simulink model "DASD_B_Project_3"  (R2025b)
settings: Solver=FixedStepAuto  StartTime=0.0  StopTime=200  FixedStep=0.01  RelTol=1e-3
values from neighbouring files (symbols this model uses):
  a = 0.923    [VehicleParameters.m]
  a_max_acc = 2.0    (= 2)    [main.m]
  a_max_dec = -3.5    [main.m]
  ABS_parameters = [lower_acc; lower_slip; higher_acc; mean_acc; rise_rate; fall_rate]    [main.m]
  b = 1.376    [VehicleParameters.m]
  CMy = 0.1    [VehicleParameters.m]
  coeff = ones(1, fir_window) / fir_window    [main.m]
  Cx = 0.33    [VehicleParameters.m]
  Cz = 0.2    [VehicleParameters.m]
  dist0 = 100    [main.m]
  eta_t = 0.93    [VehicleParameters.m]
  f0 = 0.011    [VehicleParameters.m]
  g = 9.81    [VehicleParameters.m]
  gear_vec = i_g    [main.m]
  h = 2.7    [main.m]
  hG = 0.6    [VehicleParameters.m]
  I = kp / tau_virtual    (= 1.66666666667)    [main.m]
  i_f = 3.438    [VehicleParameters.m]
  i_g = [3.909 , 2.157 , 1.48 , 1.121 , 0.897]    [VehicleParameters.m]
  Je = 0.088    [VehicleParameters.m]
  Jt = 0.05    [VehicleParameters.m]
  Jw = 0.59    [VehicleParameters.m]
  K = 2.6e-8    (= 2.6e-08)    [VehicleParameters.m]
  l = a+b    (= 2.299)    [VehicleParameters.m]
  lambda = 0.8    [main.m]
  m = 1020    [VehicleParameters.m]
  mu_vec = road_cond{choice}    [main.m]
  n_shiftdown = 200    [main.m]
  n_shiftup = 500    [main.m]
  n_vec = n_vec_set{vec_choice}    [main.m]
  omega0 = v0/Re    [main.m]
  P = kp    (= 0.333333333333)    [main.m]
  Rc = Re    (= 0.279)    [VehicleParameters.m]
  ro = 1.2    [VehicleParameters.m]
  S = 2.04    [VehicleParameters.m]
  sigma_vec = sigma    [main.m]
  startingGear = 3    [main.m]
  t_pedalAct = 0.8    [VehicleParameters.m]
  t_shifting = 0.2    [VehicleParameters.m]
  T_vec = T_vec_set{vec_choice}    [main.m]
  tau_f = 1./i_f    (= 0.290866783013)    [VehicleParameters.m]
  Tc_max = 1.2*Te_max    (= 126)    [VehicleParameters.m]
  Traction = 1    [VehicleParameters.m]
  Ts = 0.01    [main.m]
  v0 = 30    [main.m]
  v_min_acc = 5.0    (= 5)    [main.m]
  v_set_min = 7.0    (= 7)    [main.m]
libraries: simulink x29, slpidlib x1
(part 1 of 2)
settings Model: Creator=Alberto  LastModifiedBy=denni
settings OptimizationCC: ReuseModelBlockBuffer=off
settings RTWCC: GPUComputeCapability=3.5

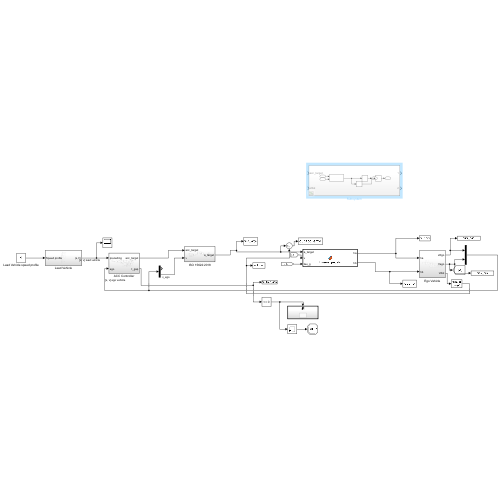
[thumbnail: Simulink's stored preview of the top-level diagram]
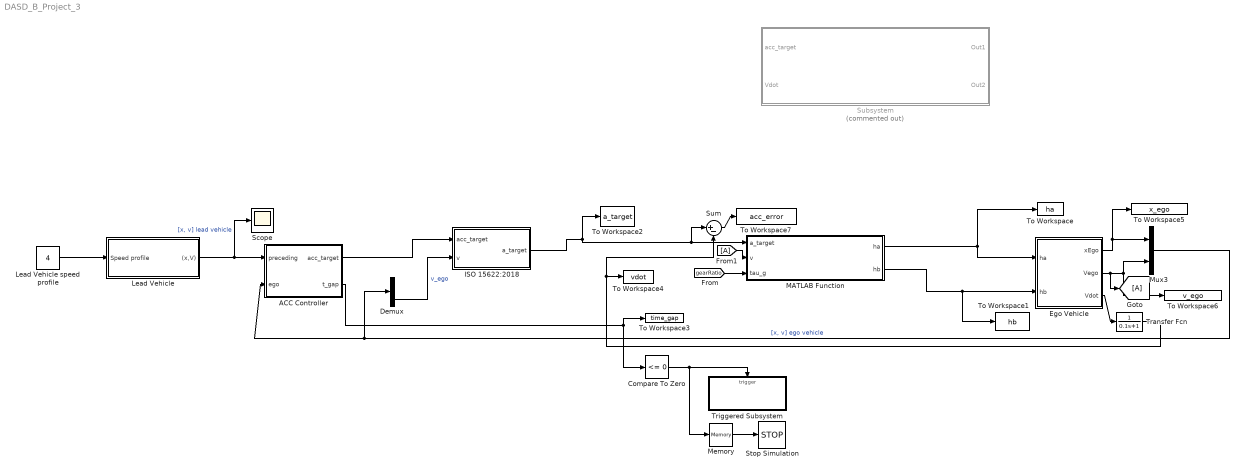
== system DASD_B_Project_3 ==
  ACC Controller : Subsystem
  Compare To Zero : simulink/Logic and Bit Operations/Compare To Zero  relop=<=  OutDataTypeStr=boolean
  Demux : Demux  Outputs=2
  Ego Vehicle : Subsystem
  From1 : From
  Goto : Goto
  ISO 15622:2018 : Subsystem
  Lead Vehicle : Subsystem
  Lead Vehicle speed profile : Constant  Value=4
  MATLAB Function : MATLAB Function  TreatAsAtomicUnit=on
  Memory : Memory
  Mux3 : Mux  Inputs=2
  Scope : Scope
      settings: ActiveDisplayYMinimum=0.0018281970394014024  ActiveDisplayYMaximum=37.912373720321341  DataLoggingVariableName=ScopeData13
  Stop Simulation : Stop
  Subsystem : Subsystem  Commented=on
  Sum : Sum  Inputs=|+-
  To Workspace : ToWorkspace  VariableName=ha  SaveFormat=Timeseries  SampleTime=-1
  To Workspace1 : ToWorkspace  VariableName=hb  SaveFormat=Timeseries  SampleTime=-1
  To Workspace2 : ToWorkspace  VariableName=a_target  SaveFormat=Timeseries  SampleTime=-1
  To Workspace3 : ToWorkspace  VariableName=time_gap  SaveFormat=Timeseries  SampleTime=-1
  To Workspace4 : ToWorkspace  VariableName=vdot  SaveFormat=Timeseries  SampleTime=-1
  To Workspace5 : ToWorkspace  VariableName=x_ego  SaveFormat=Timeseries  SampleTime=-1
  To Workspace6 : ToWorkspace  VariableName=v_ego  SaveFormat=Timeseries  SampleTime=-1
  To Workspace7 : ToWorkspace  VariableName=acc_error  SaveFormat=Timeseries  SampleTime=-1
  Transfer Fcn : TransferFcn  Denominator=[0.1 1]
  Triggered Subsystem : Subsystem  TreatAsAtomicUnit=on
  wires:
  Ego Vehicle/1(xEgo) -> To Workspace5/1, Mux3/1
  Ego Vehicle/2(Vego) -> Goto/1, To Workspace6/1, Mux3/2
  Mux3/1 -> Demux/1, ACC Controller/2(ego)  "[x, v] ego vehicle"
  Lead Vehicle/1((x,V)) -> Scope/1, ACC Controller/1(preceding)  "[x, v] lead vehicle"
  Lead Vehicle speed profile/1 -> Lead Vehicle/1(Speed profile)
  Memory/1 -> Stop Simulation/1
  Compare To Zero/1 -> Triggered Subsystem/Trigger, Memory/1
  ACC Controller/2(t_gap) -> To Workspace3/1, Compare To Zero/1
  Demux/2 -> ISO 15622:2018/2(v)  "v_ego"
  ACC Controller/1(acc_target) -> ISO 15622:2018/1(acc_target)
  ISO 15622:2018/1(a_target) -> To Workspace2/1, Sum/1, MATLAB Function/1(a_target)
  Ego Vehicle/3(Vdot) -> Transfer Fcn/1
  Transfer Fcn/1 -> To Workspace4/1, Sum/2
  [gearRatio] -> MATLAB Function/3(tau_g)
  MATLAB Function/1(ha) -> Ego Vehicle/1(ha), To Workspace/1
  MATLAB Function/2(hb) -> To Workspace1/1, Ego Vehicle/2(hb)
  Sum/1 -> To Workspace7/1
  From1/1 -> MATLAB Function/2(v)

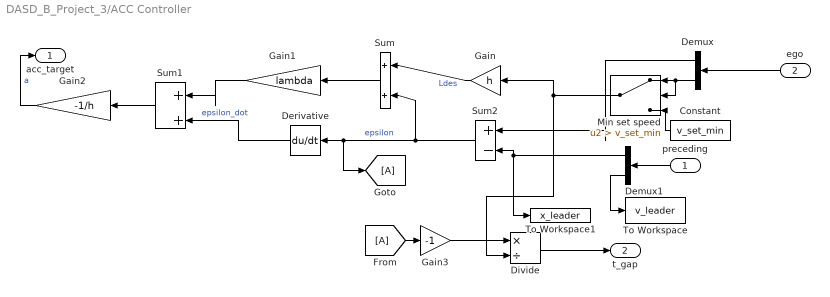
== system DASD_B_Project_3/ACC Controller ==
  preceding : Inport
  ego : Inport  Port=2
  Constant : Constant  Value=v_set_min
  Demux : Demux  Outputs=2
  Demux1 : Demux  Outputs=2
  Derivative : Derivative  CoefficientInTFapproximation=0.05
  Divide : Product  Inputs=*/
  From : From
  Gain : Gain  Gain=h
  Gain1 : Gain  Gain=lambda
  Gain2 : Gain  Gain=-1/h
  Gain3 : Gain  Gain=-1
  Goto : Goto
  Min set speed : Switch  Criteria=u2 > Threshold  Threshold=v_set_min  SaturateOnIntegerOverflow=off  InputSameDT=off
  Sum : Sum  Inputs=|++
  Sum1 : Sum  Inputs=|++
  Sum2 : Sum  Inputs=|+-
  To Workspace : ToWorkspace  VariableName=v_leader  SaveFormat=Timeseries  SampleTime=-1
  To Workspace1 : ToWorkspace  VariableName=x_leader  SaveFormat=Timeseries  SampleTime=-1
  acc_target : Outport
  t_gap : Outport  Port=2
  wires:
  Sum1/1 -> Gain2/1
  Sum/1 -> Gain1/1
  Gain2/1 -> acc_target/1  "a"
  Sum2/1 -> Sum/2, Goto/1, Derivative/1  "epsilon"
  Gain1/1 -> Sum1/1
  Gain/1 -> Sum/1  "Ldes"
  Derivative/1 -> Sum1/2  "epsilon_dot"
  ego/1 -> Demux/1
  preceding/1 -> Demux1/1
  Demux1/1 -> To Workspace1/1, Sum2/2
  Demux/1 -> Sum2/1
  Divide/1 -> t_gap/1
  From/1 -> Gain3/1
  Gain3/1 -> Divide/1
  Demux/2 -> Min set speed/2, Min set speed/1
  Min set speed/1 -> Divide/2, Gain/1
  Constant/1 -> Min set speed/3
  Demux1/2 -> To Workspace/1

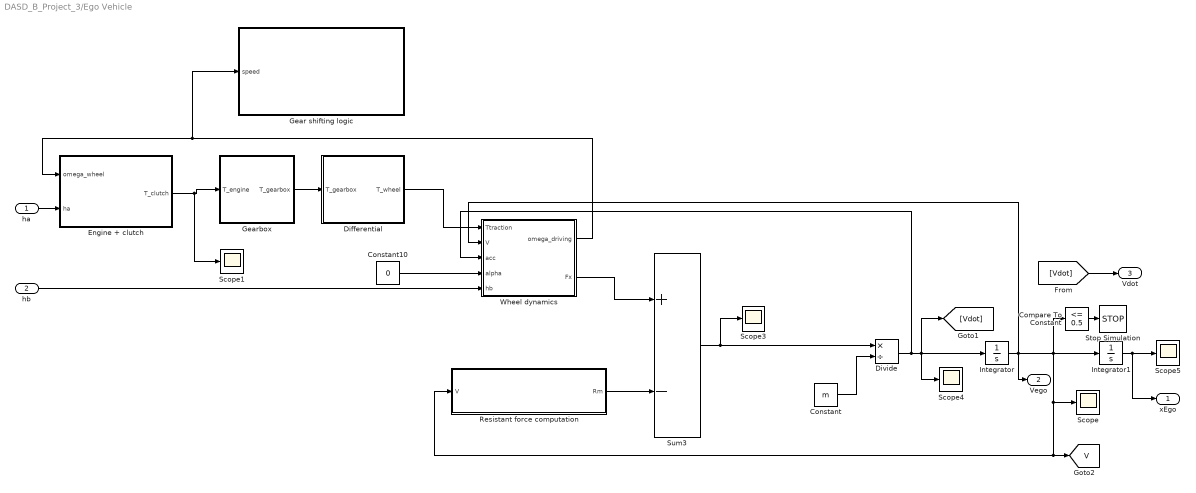
== system DASD_B_Project_3/Ego Vehicle ==
  ha : Inport
  hb : Inport  Port=2
  Compare To Constant : simulink/Logic and Bit Operations/Compare To Constant  relop=<=  const=0.5  OutDataTypeStr=boolean
  Constant : Constant  Value=m
  Constant10 : Constant  Value=0
  Differential : Subsystem
  Divide : Product  Inputs=*/
  Engine + clutch : Subsystem
  Gear shifting logic : Subsystem
  Gearbox : Subsystem
  Integrator : Integrator  InitialCondition=v0  UpperSaturationLimit=25  LowerSaturationLimit=5
  Integrator1 : Integrator
  Resistant force computation : Subsystem
  Scope{,1,3..5} (5 alike) : Scope
      Scope settings: ActiveDisplayYMinimum=2.5  ActiveDisplayYMaximum=26.27451
      Scope1 settings: ActiveDisplayYMinimum=-25.26926  ActiveDisplayYMaximum=122.58929  DataLoggingVariableName=ScopeData3
      Scope3 settings: ActiveDisplayYMinimum=-5116.83669  ActiveDisplayYMaximum=1269.91233  DataLoggingVariableName=ScopeData3
      Scope4 settings: ActiveDisplayYMinimum=-12.28873  ActiveDisplayYMaximum=11.6121  DataLoggingVariableName=ScopeData4
      Scope5 settings: ActiveDisplayYMinimum=969.20791  ActiveDisplayYMaximum=3277.1288
  Stop Simulation : Stop
  Sum3 : Sum  Inputs=+-
  Wheel dynamics : Subsystem
  xEgo : Outport
  Vego : Outport  Port=2
  Vdot : Outport  Port=3
  tag scope: V=global
  wires:
  Integrator/1 -> Wheel dynamics/2(V), Vego/1, Compare To Constant/1, [V], Resistant force computation/1(V), Scope/1, Integrator1/1
  Sum3/1 -> Scope3/1, Divide/1
  Compare To Constant/1 -> Stop Simulation/1
  Integrator1/1 -> xEgo/1, Scope5/1
  Divide/1 -> Wheel dynamics/3(acc), [Vdot], Scope4/1, Integrator/1
  Constant/1 -> Divide/2
  Resistant force computation/1(Rm) -> Sum3/2
  ha/1 -> Engine + clutch/2(ha)
  hb/1 -> Wheel dynamics/5(hb)
  Engine + clutch/1(T_clutch) -> Scope1/1, Gearbox/1(T_engine)
  Gearbox/1(T_gearbox) -> Differential/1(T_gearbox)
  Wheel dynamics/2(Fx) -> Sum3/1
  Differential/1(T_wheel) -> Wheel dynamics/1(Ttraction)
  Constant10/1 -> Wheel dynamics/4(alpha)
  Wheel dynamics/1(omega_driving) -> Gear shifting logic/1(speed), Engine + clutch/1(omega_wheel)
  [Vdot] -> Vdot/1

== system DASD_B_Project_3/ISO 15622:2018 ==
  acc_target : Inport
  v : Inport  Port=2
  Constant : Constant  Value=-3.5
  Constant1 : Constant  Value=0
  FIR filter for average acc evaluation : DiscreteFir  Coefficients=coeff
  Jerk Rate Limiter : RateLimiter  RisingSlewLimit=Inf  FallingSlewLimit=-2.5  SampleTimeMode=inherited
  Min : MinMax  Inputs=2
  Saturation : Saturate  UpperLimit=a_max_acc  LowerLimit=a_max_dec
  Scope : Scope
      settings: ActiveDisplayYMinimum=-37.751997370602687  ActiveDisplayYMaximum=46.44974892272235  DataLoggingVariableName=ScopeData12
  Switch : Switch  Criteria=u2 > Threshold  Threshold=a_max_dec  SaturateOnIntegerOverflow=off  InputSameDT=off
  Switch1 : Switch  Criteria=u2 > Threshold  Threshold=v_min_acc  SaturateOnIntegerOverflow=off  InputSameDT=off
  a_target : Outport
  wires:
  FIR filter for average acc evaluation/1 -> Switch/2
  Switch/1 -> Jerk Rate Limiter/1
  Switch1/1 -> Switch/1, FIR filter for average acc evaluation/1
  Jerk Rate Limiter/1 -> Scope/1, Saturation/1
  v/1 -> Switch1/2
  acc_target/1 -> Min/2, Switch1/1
  Min/1 -> Switch1/3
  Constant1/1 -> Min/1
  Constant/1 -> Switch/3
  Saturation/1 -> a_target/1

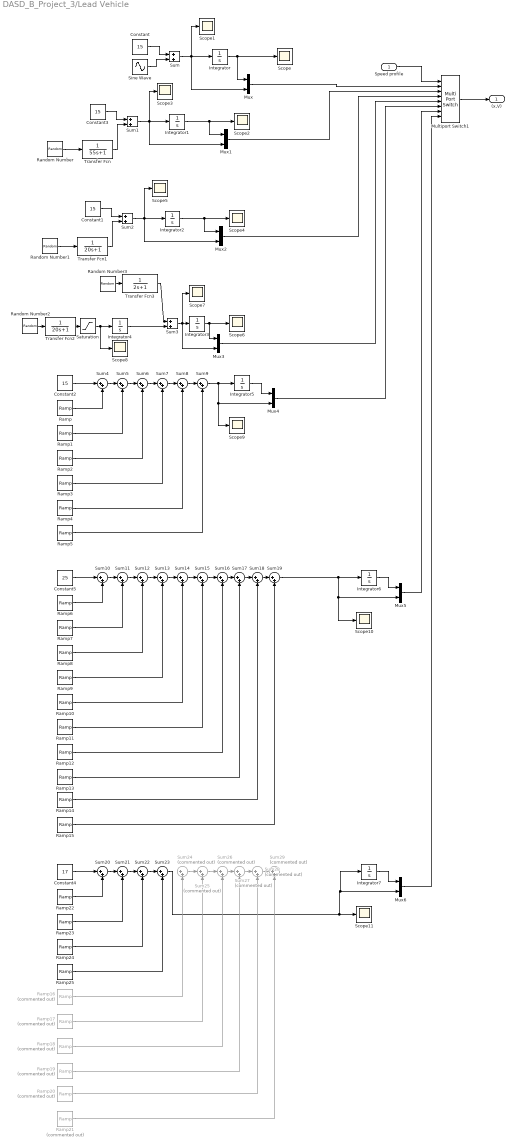
== system DASD_B_Project_3/Lead Vehicle ==
  Speed profile : Inport
  Constant{,1..3} (4 alike) : Constant  Value=15
  Constant4 : Constant  Value=17
  Constant5 : Constant  Value=25
  Integrator{,1..3,5..7} (7 alike) : Integrator  InitialCondition=dist0
  Integrator4 : Integrator  InitialCondition=15  LimitOutput=on  UpperSaturationLimit=27  LowerSaturationLimit=5
  Multiport Switch1 : MultiPortSwitch  Inputs=7  SaturateOnIntegerOverflow=off  InputSameDT=off
  Mux{,1..6} (7 alike) : Mux  Inputs=2
  Ramp : simulink/Sources/Ramp  slope=4  start=85  InitialOutput=0
  Ramp1 : simulink/Sources/Ramp  slope=-4  start=86.5  InitialOutput=0
  Ramp10 : simulink/Sources/Ramp  slope=1  start=105  InitialOutput=0
  Ramp11 : simulink/Sources/Ramp  slope=-1  start=120.3  InitialOutput=0
  Ramp12 : simulink/Sources/Ramp  slope=-15  start=150  InitialOutput=0
  Ramp13 : simulink/Sources/Ramp  slope=15  start=151.5  InitialOutput=0
  Ramp14 : simulink/Sources/Ramp  slope=8  start=165  InitialOutput=0
  Ramp15 : simulink/Sources/Ramp  slope=-8  start=167.8  InitialOutput=0
  Ramp16 : simulink/Sources/Ramp  Commented=on  slope=1  start=105  InitialOutput=0
  Ramp17 : simulink/Sources/Ramp  Commented=on  slope=-1  start=120.3  InitialOutput=0
  Ramp18 : simulink/Sources/Ramp  Commented=on  slope=-15  start=150  InitialOutput=0
  Ramp19 : simulink/Sources/Ramp  Commented=on  slope=15  start=151.5  InitialOutput=0
  Ramp2 : simulink/Sources/Ramp  slope=-12  start=150  InitialOutput=0
  Ramp20 : simulink/Sources/Ramp  Commented=on  slope=8  start=165  InitialOutput=0
  Ramp21 : simulink/Sources/Ramp  Commented=on  slope=-8  start=167.8  InitialOutput=0
  Ramp22 : simulink/Sources/Ramp  slope=-1  start=20  InitialOutput=0
  Ramp23 : simulink/Sources/Ramp  slope=1  start=30  InitialOutput=0
  Ramp24 : simulink/Sources/Ramp  slope=5  start=230  InitialOutput=0
  Ramp25 : simulink/Sources/Ramp  slope=-5  start=233  InitialOutput=0
  Ramp3 : simulink/Sources/Ramp  slope=12  start=151  InitialOutput=0
  Ramp4 : simulink/Sources/Ramp  slope=3  start=250  InitialOutput=0
  Ramp5 : simulink/Sources/Ramp  slope=-3  start=255  InitialOutput=0
  Ramp6 : simulink/Sources/Ramp  slope=-13  start=85  InitialOutput=0
  Ramp7 : simulink/Sources/Ramp  slope=13  start=86.6  InitialOutput=0
  Ramp8 : simulink/Sources/Ramp  slope=5  start=92  InitialOutput=0
  Ramp9 : simulink/Sources/Ramp  slope=-5  start=93.1  InitialOutput=0
  Random Number : RandomNumber  Variance=20  Seed=23564  SampleTime=5
  Random Number1 : RandomNumber  Variance=35  Seed=23564  SampleTime=1
  Random Number2 : RandomNumber  Variance=3  Seed=23564  SampleTime=2
  Random Number3 : RandomNumber  Variance=3  Seed=23564  SampleTime=2
  Saturation : Saturate  UpperLimit=5  LowerLimit=-5
  Scope{,1..11} (12 alike) : Scope
      Scope settings: ActiveDisplayYMinimum=62.13005  ActiveDisplayYMaximum=440.82954
      Scope1 settings: ActiveDisplayYMinimum=9.90107  ActiveDisplayYMaximum=19.94712  DataLoggingVariableName=ScopeData2
      Scope10 settings: ActiveDisplayYMinimum=-0.3125  ActiveDisplayYMaximum=27.8125  DataLoggingVariableName=ScopeData20
      Scope11 settings: ActiveDisplayYMinimum=5.125  ActiveDisplayYMaximum=23.875
      Scope2 settings: ActiveDisplayYMinimum=128.26697  ActiveDisplayYMaximum=160.50679  DataLoggingVariableName=ScopeData3
      Scope3 settings: ActiveDisplayYMinimum=13.6719  ActiveDisplayYMaximum=16.88686  DataLoggingVariableName=ScopeData4
      Scope4 settings: ActiveDisplayYMinimum=128.26697  ActiveDisplayYMaximum=160.50679  DataLoggingVariableName=ScopeData14
      Scope5 settings: ActiveDisplayYMinimum=12.15734  ActiveDisplayYMaximum=17.04494  DataLoggingVariableName=ScopeData15
      Scope6 settings: ActiveDisplayYMinimum=128.26697  ActiveDisplayYMaximum=160.50679  DataLoggingVariableName=ScopeData16
      Scope7 settings: ActiveDisplayYMinimum=-2.38071  ActiveDisplayYMaximum=32.83051  DataLoggingVariableName=ScopeData17
      Scope8 settings: ActiveDisplayYMinimum=-0.8596  ActiveDisplayYMaximum=0.81866  DataLoggingVariableName=ScopeData18
      Scope9 settings: ActiveDisplayYMinimum=7.125  ActiveDisplayYMaximum=25.875  DataLoggingVariableName=ScopeData19
  Sine Wave : Sin  Amplitude=5  SampleTime=0
  Sum{,1..3} (4 alike) : Sum
  Sum{4..23} (20 alike) : Sum  Inputs=|++
  Sum{24..29} (6 alike) : Sum  Commented=on  Inputs=|++
  Transfer Fcn : TransferFcn  Denominator=[55 1]
  Transfer Fcn1 : TransferFcn  Denominator=[20 1]
  Transfer Fcn2 : TransferFcn  Denominator=[20 1]
  Transfer Fcn3 : TransferFcn  Denominator=[2 1]
  (x,V) : Outport
  wires:
  Mux/1 -> Multiport Switch1/2
  Integrator/1 -> Scope/1, Mux/1
  Speed profile/1 -> Multiport Switch1/1
  Sum1/1 -> Integrator1/1, Mux1/2, Scope3/1
  Mux1/1 -> Multiport Switch1/3
  Transfer Fcn/1 -> Sum1/2
  Random Number/1 -> Transfer Fcn/1
  Constant/1 -> Sum/1
  Sine Wave/1 -> Sum/2
  Sum/1 -> Mux/2, Scope1/1, Integrator/1
  Integrator1/1 -> Mux1/1, Scope2/1
  Constant3/1 -> Sum1/1
  Multiport Switch1/1 -> (x,V)/1
  Constant1/1 -> Sum2/1
  Integrator2/1 -> Scope4/1, Mux2/1
  Random Number1/1 -> Transfer Fcn1/1
  Transfer Fcn1/1 -> Sum2/2
  Sum2/1 -> Integrator2/1, Scope5/1, Mux2/2
  Mux2/1 -> Multiport Switch1/4
  Mux3/1 -> Multiport Switch1/5
  Integrator4/1 -> Sum3/2
  Integrator3/1 -> Mux3/1, Scope6/1
  Saturation/1 -> Scope8/1, Integrator4/1
  Random Number2/1 -> Transfer Fcn2/1
  Transfer Fcn2/1 -> Saturation/1
  Sum3/1 -> Integrator3/1, Mux3/2, Scope7/1
  Random Number3/1 -> Transfer Fcn3/1
  Transfer Fcn3/1 -> Sum3/1
  Constant2/1 -> Sum4/1
  Ramp/1 -> Sum4/2
  Sum4/1 -> Sum5/1
  Ramp1/1 -> Sum5/2
  Sum5/1 -> Sum6/1
  Sum6/1 -> Sum7/1
  Ramp2/1 -> Sum6/2
  Ramp3/1 -> Sum7/2
  Sum7/1 -> Sum8/1
  Sum8/1 -> Sum9/1
  Ramp4/1 -> Sum8/2
  Ramp5/1 -> Sum9/2
  Sum9/1 -> Integrator5/1, Scope9/1, Mux4/2
  Integrator5/1 -> Mux4/1
  Mux4/1 -> Multiport Switch1/6
  Ramp6/1 -> Sum10/2
  Sum14/1 -> Sum15/1
  Ramp10/1 -> Sum14/2
  Sum10/1 -> Sum11/1
  Ramp9/1 -> Sum13/2
  Ramp8/1 -> Sum12/2
  Constant5/1 -> Sum10/1
  Ramp7/1 -> Sum11/2
  Sum12/1 -> Sum13/1
  Ramp11/1 -> Sum15/2
  Sum11/1 -> Sum12/1
  Sum13/1 -> Sum14/1
  Ramp13/1 -> Sum17/2
  Ramp12/1 -> Sum16/2
  Sum15/1 -> Sum16/1
  Sum16/1 -> Sum17/1
  Integrator6/1 -> Mux5/1
  Mux5/1 -> Multiport Switch1/7
  Sum17/1 -> Sum18/1
  Sum18/1 -> Sum19/1
  Ramp14/1 -> Sum18/2
  Ramp15/1 -> Sum19/2
  Sum19/1 -> Integrator6/1, Mux5/2, Scope10/1
  Sum23/1 -> Integrator7/1, Mux6/2, Scope11/1
  Sum25/1 -> Sum26/1
  Sum24/1 -> Sum25/1
  Sum28/1 -> Sum29/1
  Mux6/1 -> Multiport Switch1/8
  Ramp21/1 -> Sum29/2
  Ramp23/1 -> Sum21/2
  Ramp20/1 -> Sum28/2
  Ramp17/1 -> Sum25/2
  Ramp19/1 -> Sum27/2
  Sum20/1 -> Sum21/1
  Sum22/1 -> Sum23/1
  Constant4/1 -> Sum20/1
  Sum27/1 -> Sum28/1
  Ramp16/1 -> Sum24/2
  Integrator7/1 -> Mux6/1
  Ramp22/1 -> Sum20/2
  Ramp24/1 -> Sum22/2
  Ramp25/1 -> Sum23/2
  Ramp18/1 -> Sum26/2
  Sum26/1 -> Sum27/1
  Sum21/1 -> Sum22/1

== system DASD_B_Project_3/Subsystem ==
  acc_target : Inport
  Vdot : Inport  Port=2
  Abs : Abs  SaturateOnIntegerOverflow=off
  PI controller : Subsystem
  Saturation1 : Saturate  UpperLimit=1  LowerLimit=0
  Saturation2 : Saturate  UpperLimit=0  LowerLimit=-1
  Out1 : Outport
  Out2 : Outport  Port=2
  wires:
  Saturation1/1 -> Out1/1
  PI controller/1(a_target) -> Saturation2/1, Saturation1/1
  Saturation2/1 -> Abs/1
  Abs/1 -> Out2/1
  acc_target/1 -> PI controller/1(acc_target)
  Vdot/1 -> PI controller/2(Vdot)

== system DASD_B_Project_3/Triggered Subsystem ==
  Trigger : TriggerPort  VariantControl=(inherit)
  MATLAB Function : MATLAB Function  TreatAsAtomicUnit=on

== system DASD_B_Project_3/Ego Vehicle/Differential ==
  T_gearbox : Inport
  Gain3 : Gain  Gain=0.5*i_f
  T_wheel : Outport
  wires:
  T_gearbox/1 -> Gain3/1
  Gain3/1 -> T_wheel/1

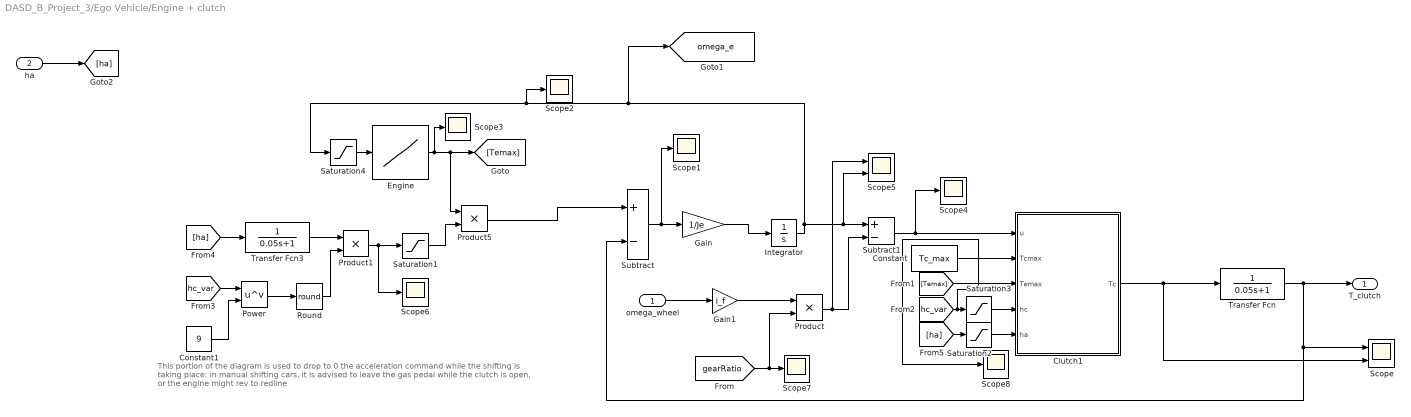
== system DASD_B_Project_3/Ego Vehicle/Engine + clutch ==
  note: This portion of the diagram is used to drop to 0 the acceleration command while the shifting is taking place: in manual shifting cars, it is advised to leave the gas pedal while the clutch is open, or the engine might rev to redline
  omega_wheel : Inport
  ha : Inport  Port=2
  Clutch1 : MATLAB Function  TreatAsAtomicUnit=on
  Constant : Constant  Value=Tc_max
  Constant1 : Constant  Value=9
  Engine : Lookup_n-D  NumberOfTableDimensions=1  BreakpointsForDimension1=n_vec  Table=T_vec  InternalRulePriority=Speed  RndMeth=Simplest
  Gain : Gain  Gain=1/Je
  Gain1 : Gain  Gain=i_f
  Integrator : Integrator  InitialCondition=omega0*i_g(5)*i_f
  Power : Math  Operator=pow
  Product : Product
  Product1 : Product
  Product5 : Product
  Round : Rounding  Operator=round
  Saturation1 : Saturate  UpperLimit=1  LowerLimit=0
  Saturation2 : Saturate  UpperLimit=1  LowerLimit=0
  Saturation3 : Saturate  UpperLimit=1  LowerLimit=0
  Saturation4 : Saturate  UpperLimit=600  LowerLimit=0
  Scope : Scope  NumInputPorts=2
      settings: ActiveDisplayYMinimum=-375  ActiveDisplayYMaximum=375  DataLoggingVariableName=ScopeData11
  Scope{1..4,6..8} (7 alike) : Scope
      Scope1 settings: ActiveDisplayYMinimum=-1.4800422611786087E+307  ActiveDisplayYMaximum=1.6444914013095649E+306  DataLoggingVariableName=ScopeData5
      Scope2 settings: ActiveDisplayYMinimum=-234.98976  ActiveDisplayYMaximum=2163.66995  DataLoggingVariableName=ScopeData6
      Scope3 settings: ActiveDisplayYMinimum=48.8411  ActiveDisplayYMaximum=110.12711  DataLoggingVariableName=ScopeData7
      Scope4 settings: ActiveDisplayYMinimum=-233.77506  ActiveDisplayYMaximum=296.88623  DataLoggingVariableName=ScopeData9
      Scope6 settings: ActiveDisplayYMinimum=-1  ActiveDisplayYMaximum=1
      Scope7 settings: ActiveDisplayYMinimum=3.85912  ActiveDisplayYMaximum=3.95022  DataLoggingVariableName=ScopeData2
      Scope8 settings: ActiveDisplayYMinimum=-0.11944  ActiveDisplayYMaximum=1.12438  DataLoggingVariableName=ScopeData2
  Scope5 : Scope  NumInputPorts=2
      settings: ActiveDisplayYMinimum=-194.18031  ActiveDisplayYMaximum=721.01575  DataLoggingVariableName=ScopeData10
  Subtract : Sum  Inputs=+-
  Subtract1 : Sum  Inputs=+-
  Transfer Fcn : TransferFcn  Denominator=[0.05 1]
  Transfer Fcn3 : TransferFcn  Denominator=[0.05 1]
  T_clutch : Outport
  tag scope: omega_e=global
  wires:
  Engine/1 -> Scope3/1, [Temax], Product5/1
  Product5/1 -> Subtract/1
  Saturation1/1 -> Product5/2
  Subtract/1 -> Scope1/1, Gain/1
  Gain/1 -> Integrator/1
  omega_wheel/1 -> Gain1/1
  Gain1/1 -> Product/1
  [gearRatio] -> Product/2, Scope7/1
  Product/1 -> Scope5/1, Subtract1/2
  Subtract1/1 -> Clutch1/1(u), Scope4/1
  Constant/1 -> Clutch1/2(Tcmax)
  [Temax] -> Clutch1/3(Temax)
  Transfer Fcn/1 -> Subtract/2, Scope/1, T_clutch/1
  Saturation3/1 -> Clutch1/4(hc)
  [hc_var] -> Scope8/1, Saturation3/1
  [ha] -> Saturation2/1
  Saturation2/1 -> Clutch1/5(ha)
  Integrator/1 -> [omega_e], Saturation4/1, Scope2/1, Scope5/2, Subtract1/1
  Transfer Fcn3/1 -> Product1/1
  Product1/1 -> Scope6/1, Saturation1/1
  Round/1 -> Product1/2
  [hc_var] -> Power/1
  Power/1 -> Round/1
  Constant1/1 -> Power/2
  Clutch1/1(Tc) -> Scope/2, Transfer Fcn/1
  Saturation4/1 -> Engine/1
  ha/1 -> [ha]
  [ha] -> Transfer Fcn3/1

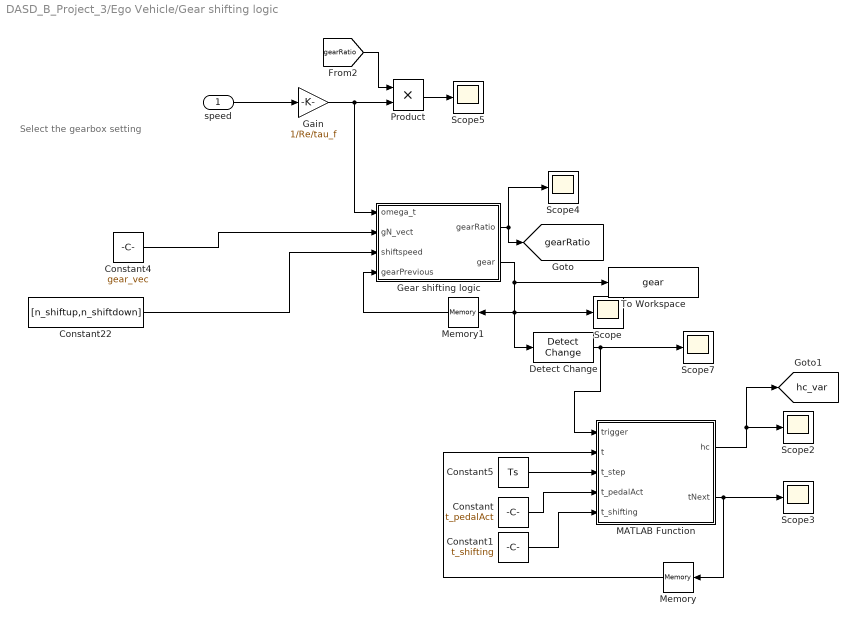
== system DASD_B_Project_3/Ego Vehicle/Gear shifting logic ==
  note: Select the gearbox setting
  speed : Inport
  Constant : Constant  Value=t_pedalAct
  Constant1 : Constant  Value=t_shifting
  Constant22 : Constant  Value=[n_shiftup,n_shiftdown]
  Constant4 : Constant  Value=gear_vec  SampleTime=Ts
  Constant5 : Constant  Value=Ts
  Detect Change : simulink/Logic and Bit Operations/Detect Change  vinit=0  OutDataTypeStr=boolean
  Gain : Gain  Gain=1/Re/tau_f
  Gear shifting logic : MATLAB Function  TreatAsAtomicUnit=on
  MATLAB Function : MATLAB Function  TreatAsAtomicUnit=on
  Memory : Memory
  Memory1 : Memory  InitialCondition=startingGear
  Product : Product
  Scope{,2..5,7} (6 alike) : Scope
      Scope settings: ActiveDisplayYMinimum=-1.6897379538383945  ActiveDisplayYMaximum=6.0412544190298609
      Scope2 settings: ActiveDisplayYMinimum=-0.11944  ActiveDisplayYMaximum=1.12438  DataLoggingVariableName=ScopeData2
      Scope3 settings: ActiveDisplayYMinimum=-0.6325  ActiveDisplayYMaximum=5.6925  DataLoggingVariableName=ScopeData3
      Scope4 settings: ActiveDisplayYMinimum=0.5205  ActiveDisplayYMaximum=4.2855  DataLoggingVariableName=ScopeData8
      Scope5 settings: ActiveDisplayYMinimum=-25.93069  ActiveDisplayYMaximum=467.45559
      Scope7 settings: ActiveDisplayYMinimum=-0.125  ActiveDisplayYMaximum=1.125  DataLoggingVariableName=ScopeData2
  To Workspace : ToWorkspace  VariableName=gear  SaveFormat=Timeseries  SampleTime=-1
  tag scope: gearRatio=global, hc_var=global
  wires:
  Gear shifting logic/1(gearRatio) -> [gearRatio], Scope4/1
  Constant22/1 -> Gear shifting logic/3(shiftspeed)
  Gear shifting logic/2(gear) -> Scope/1, Memory1/1, Detect Change/1, To Workspace/1
  Detect Change/1 -> MATLAB Function/1(trigger), Scope7/1
  MATLAB Function/2(tNext) -> Scope3/1, Memory/1
  Memory/1 -> MATLAB Function/2(t)
  MATLAB Function/1(hc) -> [hc_var], Scope2/1
  Memory1/1 -> Gear shifting logic/4(gearPrevious)
  Constant/1 -> MATLAB Function/4(t_pedalAct)
  Constant1/1 -> MATLAB Function/5(t_shifting)
  Constant5/1 -> MATLAB Function/3(t_step)
  speed/1 -> Gain/1
  Gain/1 -> Product/2, Gear shifting logic/1(omega_t)
  Constant4/1 -> Gear shifting logic/2(gN_vect)
  [gearRatio] -> Product/1
  Product/1 -> Scope5/1

== system DASD_B_Project_3/Ego Vehicle/Gearbox ==
  T_engine : Inport
  Gain2 : Gain  Gain=eta_t
  Product : Product
  T_gearbox : Outport
  wires:
  Gain2/1 -> Product/1
  T_engine/1 -> Gain2/1
  Product/1 -> T_gearbox/1
  [gearRatio] -> Product/2

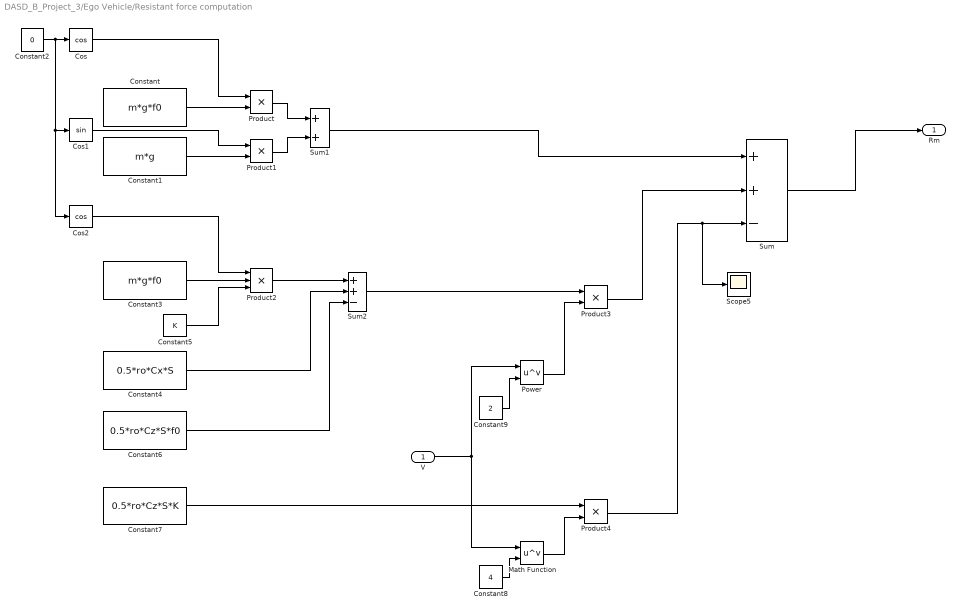
== system DASD_B_Project_3/Ego Vehicle/Resistant force computation ==
  V : Inport
  Constant : Constant  Value=m*g*f0
  Constant1 : Constant  Value=m*g
  Constant2 : Constant  Value=0
  Constant3 : Constant  Value=m*g*f0
  Constant4 : Constant  Value=0.5*ro*Cx*S
  Constant5 : Constant  Value=K
  Constant6 : Constant  Value=0.5*ro*Cz*S*f0
  Constant7 : Constant  Value=0.5*ro*Cz*S*K
  Constant8 : Constant  Value=4
  Constant9 : Constant  Value=2
  Cos : Trigonometry  Operator=cos
  Cos1 : Trigonometry
  Cos2 : Trigonometry  Operator=cos
  Math Function : Math  Operator=pow
  Power : Math  Operator=pow
  Product{,1,3..4} (4 alike) : Product
  Product2 : Product  Inputs=3
  Scope5 : Scope
      settings: ActiveDisplayYMinimum=-0.00266  ActiveDisplayYMaximum=0.02392  DataLoggingVariableName=ScopeData5
  Sum : Sum  Inputs=++-
  Sum1 : Sum
  Sum2 : Sum  Inputs=++-
  Rm : Outport
  wires:
  Constant9/1 -> Power/2
  Constant8/1 -> Math Function/2
  Constant2/1 -> Cos/1, Cos1/1, Cos2/1
  Product3/1 -> Sum/2
  Power/1 -> Product3/2
  Math Function/1 -> Product4/2
  Cos/1 -> Product/1
  Constant3/1 -> Product2/2
  V/1 -> Math Function/1, Power/1
  Constant6/1 -> Sum2/3
  Sum2/1 -> Product3/1
  Product4/1 -> Scope5/1, Sum/3
  Constant7/1 -> Product4/1
  Product/1 -> Sum1/1
  Sum1/1 -> Sum/1
  Sum/1 -> Rm/1
  Product2/1 -> Sum2/1
  Product1/1 -> Sum1/2
  Cos2/1 -> Product2/1
  Cos1/1 -> Product1/1
  Constant4/1 -> Sum2/2
  Constant/1 -> Product/2
  Constant1/1 -> Product1/2
  Constant5/1 -> Product2/3

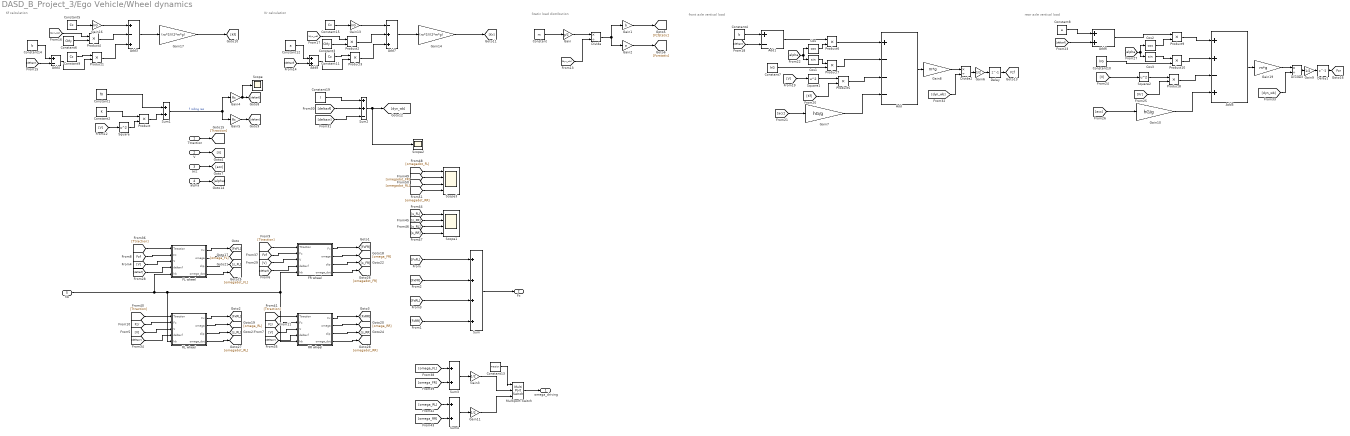
== system DASD_B_Project_3/Ego Vehicle/Wheel dynamics ==
  note: Static load distribution
  note: Kr calculation
  note: Kf calculation
  note: front axle vertical load
  note: rear axle vertical load
  Ttraction : Inport
  V : Inport  Port=2
  acc : Inport  Port=3
  alpha : Inport  Port=4
  hb : Inport  Port=5
  Add : Sum  Inputs=+---
  Add1 : Sum  Inputs=+-
  Add3 : Sum  Inputs=+-+
  Add4 : Sum  Inputs=+-
  Add5 : Sum  Inputs=++-+
  Add6 : Sum
  Add7 : Sum  Inputs=-++
  Add8 : Sum
  Constant : Constant  Value=m
  Constant1 : Constant  Value=f0
  Constant10 : Constant  Value=hG
  Constant11 : Constant  Value=Cz
  Constant12 : Constant  Value=a
  Constant13 : Constant  Value=Traction
  Constant14 : Constant  Value=b
  Constant15 : Constant  Value=Cx
  Constant19 : Constant  Value=l
  Constant2 : Constant  Value=K
  Constant3 : Constant  Value=CMy
  Constant4 : Constant  Value=b
  Constant5 : Constant  Value=Cx
  Constant6 : Constant  Value=CMy
  Constant7 : Constant  Value=hG
  Constant8 : Constant  Value=a
  Constant9 : Constant  Value=Cz
  Cos : Trigonometry  Operator=cos
  Cos1 : Trigonometry
  Cos2 : Trigonometry  Operator=cos
  Cos3 : Trigonometry
  Delay : Delay  DelayLength=1  InitialCondition=m*g*b/l/2
  Delay1 : Delay  DelayLength=1  InitialCondition=m*g*a/l/2
  Divide : Product  Inputs=*/
  Divide2 : Product  Inputs=*/
  Divide3 : Product  Inputs=*/
  FL wheel : Subsystem
  FR wheel : Subsystem
  Gain : Gain  Gain=g/2
  Gain1 : Gain  Gain=b
  Gain10 : Gain  Gain=hG/g
  Gain{3,6,9,11} (4 alike) : Gain  Gain=1/2
  Gain13 : Gain  Gain=hG
  Gain14 : Gain  Gain=(ro*S)/(2*m*g)
  Gain16 : Gain  Gain=hG
  Gain17 : Gain  Gain=(ro*S)/(2*m*g)
  Gain19 : Gain  Gain=m*g
  Gain2 : Gain  Gain=a
  Gain4 : Gain  Gain=Rc
  Gain5 : Gain  Gain=Rc
  Gain7 : Gain  Gain=hG/g
  Gain8 : Gain  Gain=m*g
  Multiport Switch : MultiPortSwitch  Inputs=2  SaturateOnIntegerOverflow=off  InputSameDT=off
  Product{,1..10} (11 alike) : Product
  RL wheel : Subsystem
  RR wheel : Subsystem
  Scope : Scope
      settings: ActiveDisplayYMinimum=0.003067  ActiveDisplayYMaximum=0.003086  DataLoggingVariableName=ScopeData2
  Scope1 : Scope  NumInputPorts=4
      settings: ActiveDisplayYMinimum=-0.81631  ActiveDisplayYMaximum=0.66165  DataLoggingVariableName=slip
  Scope2 : Scope
      settings: ActiveDisplayYMinimum=1.299  ActiveDisplayYMaximum=3.299  DataLoggingVariableName=ScopeData4
  Scope3 : Scope  NumInputPorts=4
      settings: ActiveDisplayYMinimum=-0.81631  ActiveDisplayYMaximum=0.66165  DataLoggingVariableName=omegadot
  Square : Math  Operator=square
  Square1 : Math  Operator=square
  Square2 : Math  Operator=square
  Sum : Sum  Inputs=++++
  Sum1 : Sum
  Sum2 : Sum  Inputs=++-
  Sum3 : Sum
  Sum4 : Sum
  omega_driving : Outport
  Fx : Outport  Port=2
  tag scope: Fzf=global, Fzr=global
  wires:
  FL wheel/1(Fx) -> [FxFL]
  [V] -> RR wheel/3(V)
  [FxRL] -> Sum/3
  V/1 -> [V]
  Sum/1 -> Fx/1
  RR wheel/1(Fx) -> [FxRR]
  [FxRR] -> Sum/4
  [FxFL] -> Sum/1
  FR wheel/1(Fx) -> [FxFR]
  [FxFR] -> Sum/2
  [V] -> FL wheel/3(V)
  [V] -> RL wheel/3(V)
  RL wheel/1(Fx) -> [FxRL]
  [Fzf] -> FL wheel/2(Fz)
  Constant/1 -> Gain/1
  Gain1/1 -> [Fzfstatic]
  Gain2/1 -> [Fzrstatic]
  [Fzr] -> RL wheel/2(Fz)
  [Fzr] -> RR wheel/2(Fz)
  acc/1 -> [acc]
  [V] -> Square/1
  Constant2/1 -> Product/1
  Square/1 -> Product/2
  Constant1/1 -> Sum1/1
  Product/1 -> Sum1/2
  Sum1/1 -> Gain5/1, Gain4/1  "f rolling res"
  Gain4/1 -> Scope/1, [deltaxf]
  Gain5/1 -> [deltaxr]
  Constant19/1 -> Sum2/1
  [deltaxr] -> Sum2/3
  Sum2/1 -> Scope2/1, [dyn_wb]
  [deltaxf] -> Sum2/2
  Gain/1 -> Divide/1
  [dyn_wb] -> Divide/2
  Divide/1 -> Gain2/1, Gain1/1
  Add4/1 -> Product1/2
  Gain17/1 -> [Kf]
  Product1/1 -> Add3/3
  Product3/1 -> Add7/3
  Constant5/1 -> Gain16/1
  Add8/1 -> Product3/2
  Constant12/1 -> Add8/1
  Constant15/1 -> Gain13/1
  Product2/1 -> Add7/2
  Product4/1 -> Add3/2
  Add3/1 -> Gain17/1
  Constant9/1 -> Product1/1
  Constant11/1 -> Product3/1
  [deltaxr] -> Add4/2
  Add7/1 -> Gain14/1
  Gain14/1 -> [Kr]
  [deltaxf] -> Add8/2
  Gain13/1 -> Add7/1
  Gain16/1 -> Add3/1
  Constant14/1 -> Add4/1
  Constant6/1 -> Product4/2
  [dyn_wb] -> Product4/1
  Constant3/1 -> Product2/2
  [dyn_wb] -> Product2/1
  Product5/1 -> Add/3
  Gain7/1 -> Add/4
  Square1/1 -> Product5/1
  Constant4/1 -> Add1/1
  [Kf] -> Product5/2
  Product7/1 -> Add/2
  Add1/1 -> Product6/1
  Constant7/1 -> Product7/2
  [dyn_wb] -> Divide2/2
  [V] -> Square1/1
  [acc] -> Gain7/1
  Gain8/1 -> Divide2/1
  Product6/1 -> Add/1
  Add/1 -> Gain8/1
  [deltaxr] -> Add1/2
  Cos/1 -> Product6/2
  Cos1/1 -> Product7/1
  alpha/1 -> [alpha]
  [alpha] -> Cos/1, Cos1/1
  Divide2/1 -> Gain6/1
  [V] -> Square2/1
  [acc] -> Gain10/1
  Constant10/1 -> Product10/2
  Add5/1 -> Gain19/1
  Constant8/1 -> Add6/1
  Product9/1 -> Add5/1
  [dyn_wb] -> Divide3/2
  Add6/1 -> Product9/1
  Square2/1 -> Product8/1
  Product8/1 -> Add5/3
  [Kr] -> Product8/2
  Gain19/1 -> Divide3/1
  Gain10/1 -> Add5/4
  Product10/1 -> Add5/2
  [deltaxf] -> Add6/2
  [alpha] -> Cos2/1, Cos3/1
  Cos2/1 -> Product9/2
  Cos3/1 -> Product10/1
  Divide3/1 -> Gain9/1
  Gain6/1 -> Delay/1
  Delay/1 -> [Fzf]
  Gain9/1 -> Delay1/1
  [deltaxf] -> FL wheel/4(deltaxf)
  [deltaxr] -> RL wheel/4(deltaxf)
  [deltaxr] -> RR wheel/4(deltaxf)
  Delay1/1 -> [Fzr]
  Ttraction/1 -> [Ttraction]
  [Ttraction] -> FL wheel/1(Ttraction)
  [Ttraction] -> FR wheel/1(Ttraction)
  [V] -> FR wheel/3(V)
  [deltaxf] -> FR wheel/4(deltaxf)
  [Fzf] -> FR wheel/2(Fz)
  FL wheel/2(omega) -> [omega_FL]
  FR wheel/2(omega) -> [omega_FR]
  [omega_FL] -> Sum3/1
  [omega_FR] -> Sum3/2
  Sum3/1 -> Gain3/1
  [Ttraction] -> RL wheel/1(Ttraction)
  RL wheel/2(omega) -> [omega_RL]
  [Ttraction] -> RR wheel/1(Ttraction)
  RR wheel/2(omega) -> [omega_RR]
  Sum4/1 -> Gain11/1
  [omega_RR] -> Sum4/2
  [omega_RL] -> Sum4/1
  Gain3/1 -> Multiport Switch/2
  Gain11/1 -> Multiport Switch/3
  Constant13/1 -> Multiport Switch/1
  Multiport Switch/1 -> omega_driving/1
  FL wheel/3(slip) -> [s_FL]
  FR wheel/3(slip) -> [s_FR]
  RL wheel/3(slip) -> [s_RL]
  RR wheel/3(slip) -> [s_RR]
  [s_FL] -> Scope1/1
  [s_FR] -> Scope1/2
  [s_RL] -> Scope1/3
  [s_RR] -> Scope1/4
  FL wheel/4(omega_dot) -> [omegadot_FL]
  FR wheel/4(omega_dot) -> [omegadot_FR]
  RL wheel/4(omega_dot) -> [omegadot_RL]
  RR wheel/4(omega_dot) -> [omegadot_RR]
  [omegadot_RR] -> Scope3/4
  [omegadot_RL] -> Scope3/3
  [omegadot_FR] -> Scope3/2
  [omegadot_FL] -> Scope3/1
  hb/1 -> RR wheel/5(hb), FR wheel/5(hb), RL wheel/5(hb), FL wheel/5(hb)

== system DASD_B_Project_3/Subsystem/PI controller ==
  acc_target : Inport
  Vdot : Inport  Port=2
  Add : Sum  Inputs=+-
  PID Controller : slpidlib/PID Controller  Controller=PI  Form=Parallel  TimeDomain=Continuous-time  UseExternalTs=off  SampleTime=Ts  IntegratorMethod=Forward Euler  FilterMethod=Forward Euler  ControllerParametersSource=internal  P=P  I=I  UseKiTs=off  D=0  UseExternalDerivativeSource=off  N=100  UseFilter=on  TunerSelectOption=Transfer Function Based (PID Tuner App)  InitialConditionSource=internal  InitialConditionForIntegrator=0  InitialConditionForFilter=0  DifferentiatorICPrevScaledInput=0  ExternalReset=none  TrackingMode=off  Kt=1  LimitOutput=on  SatLimitsSource=internal  UpperSaturationLimit=1  LowerSaturationLimit=-1  LinearizeAsGain=on  AntiWindupMode=clamping  Kb=1  LimitIntegrator=off  UpperIntegratorSaturationLimit=inf  LowerIntegratorSaturationLimit=-inf  POutMin=[]  POutMax=[]  IOutMin=[]  IOutMax=[]  DOutMin=[]  DOutMax=[]  NOutMin=[]  NOutMax=[]  SumOutMin=[]  SumOutMax=[]  SaturationOutMin=[]  SaturationOutMax=[]  PParamMin=[]  PParamMax=[]  IParamMin=[]  IParamMax=[]  DParamMin=[]  DParamMax=[]  NParamMin=[]  NParamMax=[]  KbParamMin=[]  KbParamMax=[]  KtParamMin=[]  KtParamMax=[]  KbOutMin=[]  KbOutMax=[]  KtOutMin=[]  KtOutMax=[]  IntegratorOutMin=[]  IntegratorOutMax=[]  FilterOutMin=[]  FilterOutMax=[]  SumI1OutMin=[]  SumI1OutMax=[]  SumI2OutMin=[]  SumI2OutMax=[]  SumI3OutMin=[]  SumI3OutMax=[]  SumI4OutMin=[]  SumI4OutMax=[]  SumDOutMin=[]  SumDOutMax=[]  DifferentiatorOutMin=[]  DifferentiatorOutMax=[]  FilterDiffOutCoefMin=[]  FilterDiffOutCoefMax=[]  ReciprocalOutMin=[]  ReciprocalOutMax=[]  SumDenOutMin=[]  SumDenOutMax=[]  SumNumOutMin=[]  SumNumOutMax=[]  DivideOutMin=[]  DivideOutMax=[]  UdiffTsProdOutMin=[]  UdiffTsProdOutMax=[]  NTsProdOutMin=[]  NTsProdOutMax=[]  UintegralTsProdOutMin=[]  UintegralTsProdOutMax=[]  UngainTsProdOutMin=[]  UngainTsProdOutMax=[]  ClampingZeroOutDataTypeStr=Inherit: Inherit via back propagation  ClampingZeroOutMin=[]  ClampingZeroOutMax=[]  FilterDenConstantOutDataTypeStr=Inherit: Inherit via back propagation  FilterDenConstantOutMin=[]  FilterDenConstantOutMax=[]  PCopyOutDataTypeStr=Inherit: Inherit via back propagation  PCopyOutMin=[]  PCopyOutMax=[]  NCopyOutDataTypeStr=Inherit: Inherit via back propagation  NCopyOutMin=[]  NCopyOutMax=[]  IntegratorContinuousStateAttributes=''  IntegratorStateMustResolveToSignalObject=off  IntegratorRTWStateStorageClass=Auto  FilterContinuousStateAttributes=''  FilterStateMustResolveToSignalObject=off  FilterRTWStateStorageClass=Auto  ParallelPVariant=InternalParameters  IdealPVariant=Disabled  IVariant=InternalParameters  DVariant=Disabled  IntegratorVariant=Continuous  SatVariant=Enabled  AWVariant=ContClampingParallel  PCopyVariant=Disabled  TRVariant=Disabled  FdbkBlocksVariant=Forward  IdealPFdbkVariant=Disabled  SatFdbkVariant=Disabled  DerivativeFilterVariant=Disabled  NVariant=Disabled  NCopyVariant=Disabled_SignalSpec  FilterICVariant=Disabled  IntegratorICVariant=InternalICs  ExternalResetVariant=Disabled  TRSumVariant=Passthrough  SumFdbkVariant=Disabled  SumVariant=Sum_PI  TsampFilterVariant=InternalTs  TsampNgainVariant=Passthrough  TsampIntegralVariant=Disabled_SignalSpec  ExternalSaturationOutDataTypeStr=Inherit: Same as second input  DerivativeSourceVariant=Disabled  PreIntVariant=InternalPreInt
  To Workspace5 : ToWorkspace  VariableName=acc_error  SaveFormat=Timeseries  SampleTime=-1
  a_target : Outport
  wires:
  Add/1 -> To Workspace5/1, PID Controller/1  "acc error"
  acc_target/1 -> Add/1
  PID Controller/1 -> a_target/1
  Vdot/1 -> Add/2

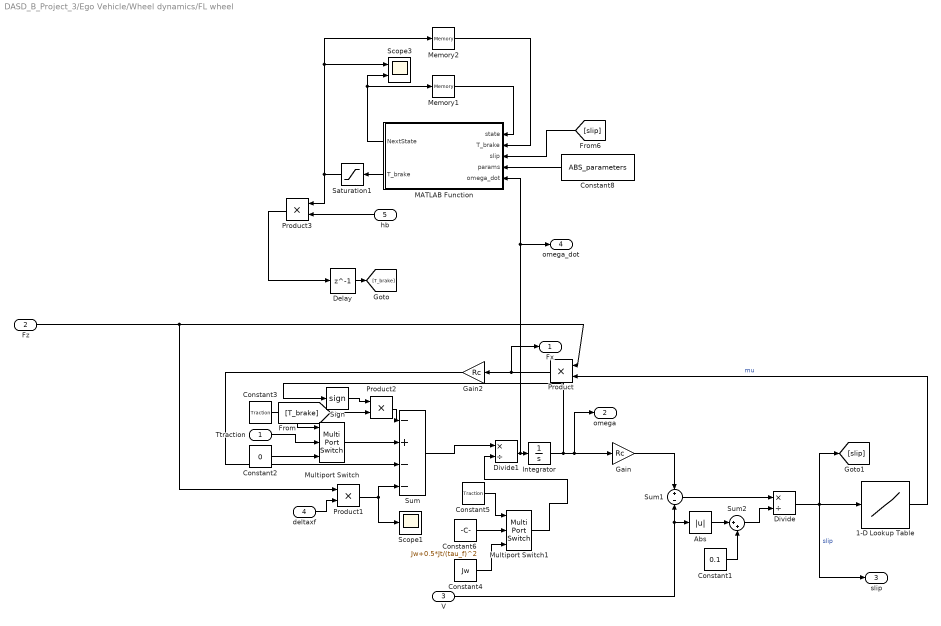
== system DASD_B_Project_3/Ego Vehicle/Wheel dynamics/FL wheel ==
  Ttraction : Inport
  Fz : Inport  Port=2
  V : Inport  Port=3
  deltaxf : Inport  Port=4
  hb : Inport  Port=5
  1-D Lookup Table : Lookup_n-D  NumberOfTableDimensions=1  BreakpointsForDimension1=sigma_vec  Table=mu_vec  InternalRulePriority=Speed  RndMeth=Simplest
  Abs : Abs  SaturateOnIntegerOverflow=off
  Constant1 : Constant  Value=0.1
  Constant2 : Constant  Value=0
  Constant3 : Constant  Value=Traction
  Constant4 : Constant  Value=Jw
  Constant5 : Constant  Value=Traction
  Constant6 : Constant  Value=Jw+0.5*Jt/(tau_f)^2
  Constant8 : Constant  Value=ABS_parameters
  Delay : Delay  DelayLength=1
  Divide : Product  Inputs=*/
  Divide1 : Product  Inputs=*/
  Gain : Gain  Gain=Rc
  Gain2 : Gain  Gain=Rc
  Integrator : Integrator  InitialCondition=omega0
  MATLAB Function : MATLAB Function  TreatAsAtomicUnit=on
  Memory1 : Memory  InitialCondition=1
  Memory2 : Memory
  Multiport Switch : MultiPortSwitch  Inputs=2  SaturateOnIntegerOverflow=off  InputSameDT=off
  Multiport Switch1 : MultiPortSwitch  Inputs=2  SaturateOnIntegerOverflow=off  InputSameDT=off
  Product{,1..3} (4 alike) : Product
  Saturation1 : Saturate  UpperLimit=1500  LowerLimit=0
  Scope1 : Scope
      settings: ActiveDisplayYMinimum=4.6511  ActiveDisplayYMaximum=15.35009  DataLoggingVariableName=ScopeData8
  Scope3 : Scope  NumInputPorts=2
      settings: ActiveDisplayYMinimum=0.07603  ActiveDisplayYMaximum=3.82977
  Sign : Signum
  Sum : Sum  Inputs=-+--
  Sum1 : Sum  Inputs=+-
  Sum2 : Sum  Inputs=|++
  Fx : Outport
  omega : Outport  Port=2
  slip : Outport  Port=3
  omega_dot : Outport  Port=4
  wires:
  Gain/1 -> Sum1/1
  Gain2/1 -> Sum/3
  V/1 -> Abs/1, Sum1/2
  Product/1 -> Fx/1, Gain2/1
  1-D Lookup Table/1 -> Product/2  "mu"
  Integrator/1 -> Sign/1, omega/1, Gain/1
  Sum1/1 -> Divide/1
  Divide/1 -> slip/1, [slip], 1-D Lookup Table/1  "slip"
  Fz/1 -> Product/1, Product1/1
  Sum2/1 -> Divide/2
  Abs/1 -> Sum2/1
  Constant1/1 -> Sum2/2
  deltaxf/1 -> Product1/2
  Product1/1 -> Sum/4, Scope1/1
  Multiport Switch/1 -> Sum/2
  Constant2/1 -> Multiport Switch/3
  Ttraction/1 -> Multiport Switch/2
  Constant3/1 -> Multiport Switch/1
  Constant5/1 -> Multiport Switch1/1
  Multiport Switch1/1 -> Divide1/2
  Sum/1 -> Divide1/1
  Constant4/1 -> Multiport Switch1/3
  Constant6/1 -> Multiport Switch1/2
  Sign/1 -> Product2/1
  [T_brake] -> Product2/2
  Product2/1 -> Sum/1
  Saturation1/1 -> Memory2/1, Scope3/1, Product3/1
  MATLAB Function/2(T_brake) -> Saturation1/1
  Memory2/1 -> MATLAB Function/2("T_brake ")
  [slip] -> MATLAB Function/3(slip)
  Constant8/1 -> MATLAB Function/4(params)
  Memory1/1 -> MATLAB Function/1(state)
  MATLAB Function/1(NextState) -> Memory1/1, Scope3/2
  Divide1/1 -> omega_dot/1, MATLAB Function/5(omega_dot), Integrator/1
  Delay/1 -> [T_brake]
  hb/1 -> Product3/2
  Product3/1 -> Delay/1

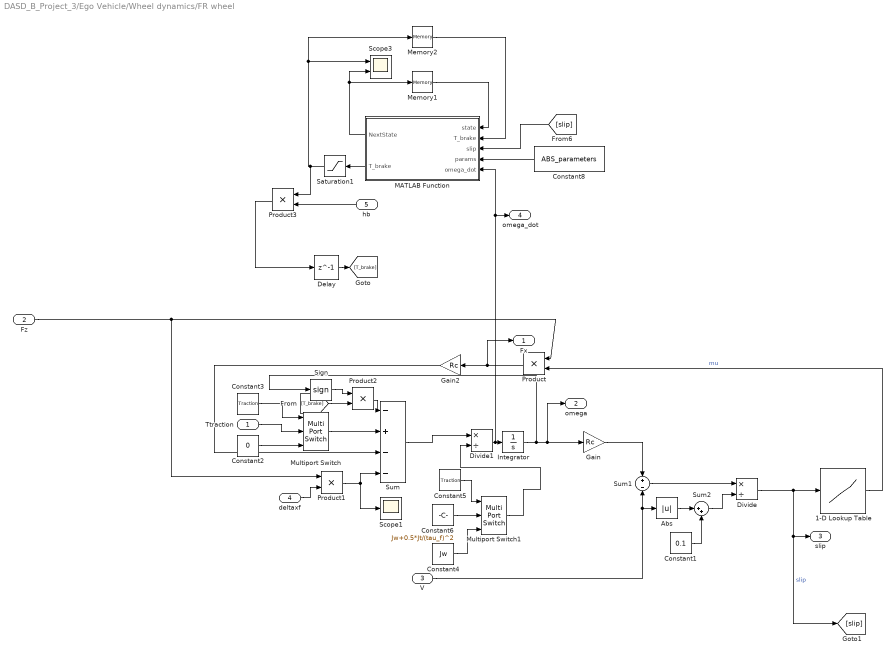
== system DASD_B_Project_3/Ego Vehicle/Wheel dynamics/FR wheel ==
  Ttraction : Inport
  Fz : Inport  Port=2
  V : Inport  Port=3
  deltaxf : Inport  Port=4
  hb : Inport  Port=5
  1-D Lookup Table : Lookup_n-D  NumberOfTableDimensions=1  BreakpointsForDimension1=sigma_vec  Table=mu_vec  InternalRulePriority=Speed  RndMeth=Simplest
  Abs : Abs  SaturateOnIntegerOverflow=off
  Constant1 : Constant  Value=0.1
  Constant2 : Constant  Value=0
  Constant3 : Constant  Value=Traction
  Constant4 : Constant  Value=Jw
  Constant5 : Constant  Value=Traction
  Constant6 : Constant  Value=Jw+0.5*Jt/(tau_f)^2
  Constant8 : Constant  Value=ABS_parameters
  Delay : Delay  DelayLength=1
  Divide : Product  Inputs=*/
  Divide1 : Product  Inputs=*/
  Gain : Gain  Gain=Rc
  Gain2 : Gain  Gain=Rc
  Integrator : Integrator  InitialCondition=omega0
  MATLAB Function : MATLAB Function  TreatAsAtomicUnit=on
  Memory1 : Memory  InitialCondition=1
  Memory2 : Memory
  Multiport Switch : MultiPortSwitch  Inputs=2  SaturateOnIntegerOverflow=off  InputSameDT=off
  Multiport Switch1 : MultiPortSwitch  Inputs=2  SaturateOnIntegerOverflow=off  InputSameDT=off
  Product{,1..3} (4 alike) : Product
  Saturation1 : Saturate  UpperLimit=1500  LowerLimit=0
  Scope1 : Scope
      settings: ActiveDisplayYMinimum=4.36579  ActiveDisplayYMaximum=14.13838  DataLoggingVariableName=ScopeData8
  Scope3 : Scope  NumInputPorts=2
      settings: ActiveDisplayYMinimum=0.07603  ActiveDisplayYMaximum=3.82977  DataLoggingVariableName=ScopeData2
  Sign : Signum
  Sum : Sum  Inputs=-+--
  Sum1 : Sum  Inputs=+-
  Sum2 : Sum  Inputs=|++
  Fx : Outport
  omega : Outport  Port=2
  slip : Outport  Port=3
  omega_dot : Outport  Port=4
  wires:
  Product2/1 -> Sum/1
  [T_brake] -> Product2/2
  Sign/1 -> Product2/1
  Constant6/1 -> Multiport Switch1/2
  Constant4/1 -> Multiport Switch1/3
  Sum/1 -> Divide1/1
  Multiport Switch1/1 -> Divide1/2
  Constant5/1 -> Multiport Switch1/1
  Constant3/1 -> Multiport Switch/1
  Ttraction/1 -> Multiport Switch/2
  Constant2/1 -> Multiport Switch/3
  Multiport Switch/1 -> Sum/2
  Product1/1 -> Scope1/1, Sum/4
  deltaxf/1 -> Product1/2
  Constant1/1 -> Sum2/2
  Abs/1 -> Sum2/1
  Sum2/1 -> Divide/2
  Fz/1 -> Product1/1, Product/1
  Divide/1 -> [slip], slip/1, 1-D Lookup Table/1  "slip"
  Sum1/1 -> Divide/1
  Integrator/1 -> Gain/1, omega/1, Sign/1
  1-D Lookup Table/1 -> Product/2  "mu"
  Product/1 -> Gain2/1, Fx/1
  V/1 -> Sum1/2, Abs/1
  Gain2/1 -> Sum/3
  Gain/1 -> Sum1/1
  Divide1/1 -> omega_dot/1, MATLAB Function/5(omega_dot), Integrator/1
  Memory2/1 -> MATLAB Function/2("T_brake ")
  MATLAB Function/2(T_brake) -> Saturation1/1
  Constant8/1 -> MATLAB Function/4(params)
  Memory1/1 -> MATLAB Function/1(state)
  MATLAB Function/1(NextState) -> Memory1/1, Scope3/2
  [slip] -> MATLAB Function/3(slip)
  Saturation1/1 -> Product3/1, Memory2/1, Scope3/1
  Product3/1 -> Delay/1
  Delay/1 -> [T_brake]
  hb/1 -> Product3/2

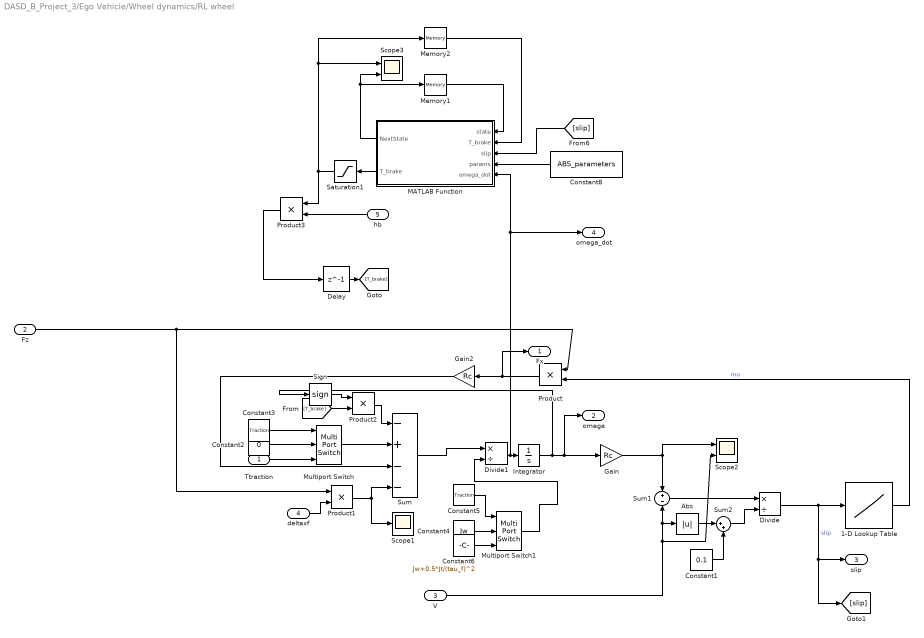
== system DASD_B_Project_3/Ego Vehicle/Wheel dynamics/RL wheel ==
  Ttraction : Inport
  Fz : Inport  Port=2
  V : Inport  Port=3
  deltaxf : Inport  Port=4
  hb : Inport  Port=5
  1-D Lookup Table : Lookup_n-D  NumberOfTableDimensions=1  BreakpointsForDimension1=sigma_vec  Table=mu_vec  InternalRulePriority=Speed  RndMeth=Simplest
  Abs : Abs  SaturateOnIntegerOverflow=off
  Constant1 : Constant  Value=0.1
  Constant2 : Constant  Value=0
  Constant3 : Constant  Value=Traction
  Constant4 : Constant  Value=Jw
  Constant5 : Constant  Value=Traction
  Constant6 : Constant  Value=Jw+0.5*Jt/(tau_f)^2
  Constant8 : Constant  Value=ABS_parameters
  Delay : Delay  DelayLength=1
  Divide : Product  Inputs=*/
  Divide1 : Product  Inputs=*/
  Gain : Gain  Gain=Rc
  Gain2 : Gain  Gain=Rc
  Integrator : Integrator  InitialCondition=omega0
  MATLAB Function : MATLAB Function  TreatAsAtomicUnit=on
  Memory1 : Memory  InitialCondition=1
  Memory2 : Memory
  Multiport Switch : MultiPortSwitch  Inputs=2  SaturateOnIntegerOverflow=off  InputSameDT=off
  Multiport Switch1 : MultiPortSwitch  Inputs=2  SaturateOnIntegerOverflow=off  InputSameDT=off
  Product{,1..3} (4 alike) : Product
  Saturation1 : Saturate  UpperLimit=1500  LowerLimit=0
  Scope1 : Scope
      settings: ActiveDisplayYMinimum=4.59074  ActiveDisplayYMaximum=6.6088  DataLoggingVariableName=ScopeData8
  Scope2 : Scope  NumInputPorts=2
      settings: ActiveDisplayYMinimum=-5.62229  ActiveDisplayYMaximum=50.6247  DataLoggingVariableName=ScopeData6
  Scope3 : Scope  NumInputPorts=2
      settings: ActiveDisplayYMinimum=0.07603  ActiveDisplayYMaximum=3.82977  DataLoggingVariableName=ScopeData3
  Sign : Signum
  Sum : Sum  Inputs=-+--
  Sum1 : Sum  Inputs=+-
  Sum2 : Sum  Inputs=|++
  Fx : Outport
  omega : Outport  Port=2
  slip : Outport  Port=3
  omega_dot : Outport  Port=4
  wires:
  Gain/1 -> Sum1/1, Scope2/1
  Gain2/1 -> Sum/3
  V/1 -> Sum1/2, Abs/1, Scope2/2
  Product/1 -> Fx/1, Gain2/1
  1-D Lookup Table/1 -> Product/2  "mu"
  Integrator/1 -> Sign/1, omega/1, Gain/1
  Sum1/1 -> Divide/1
  Divide/1 -> [slip], slip/1, 1-D Lookup Table/1  "slip"
  Fz/1 -> Product/1, Product1/1
  Sum2/1 -> Divide/2
  Abs/1 -> Sum2/1
  Constant1/1 -> Sum2/2
  deltaxf/1 -> Product1/2
  Product1/1 -> Sum/4, Scope1/1
  Multiport Switch/1 -> Sum/2
  Constant3/1 -> Multiport Switch/1
  Constant5/1 -> Multiport Switch1/1
  Multiport Switch1/1 -> Divide1/2
  Sum/1 -> Divide1/1
  Constant6/1 -> Multiport Switch1/3
  Constant4/1 -> Multiport Switch1/2
  Constant2/1 -> Multiport Switch/2
  Ttraction/1 -> Multiport Switch/3
  Product2/1 -> Sum/1
  Sign/1 -> Product2/1
  [T_brake] -> Product2/2
  Divide1/1 -> omega_dot/1, MATLAB Function/5(omega_dot), Integrator/1
  Memory2/1 -> MATLAB Function/2("T_brake ")
  MATLAB Function/2(T_brake) -> Saturation1/1
  Constant8/1 -> MATLAB Function/4(params)
  Memory1/1 -> MATLAB Function/1(state)
  MATLAB Function/1(NextState) -> Memory1/1, Scope3/2
  [slip] -> MATLAB Function/3(slip)
  Saturation1/1 -> Memory2/1, Scope3/1, Product3/1
  Product3/1 -> Delay/1
  Delay/1 -> [T_brake]
  hb/1 -> Product3/2

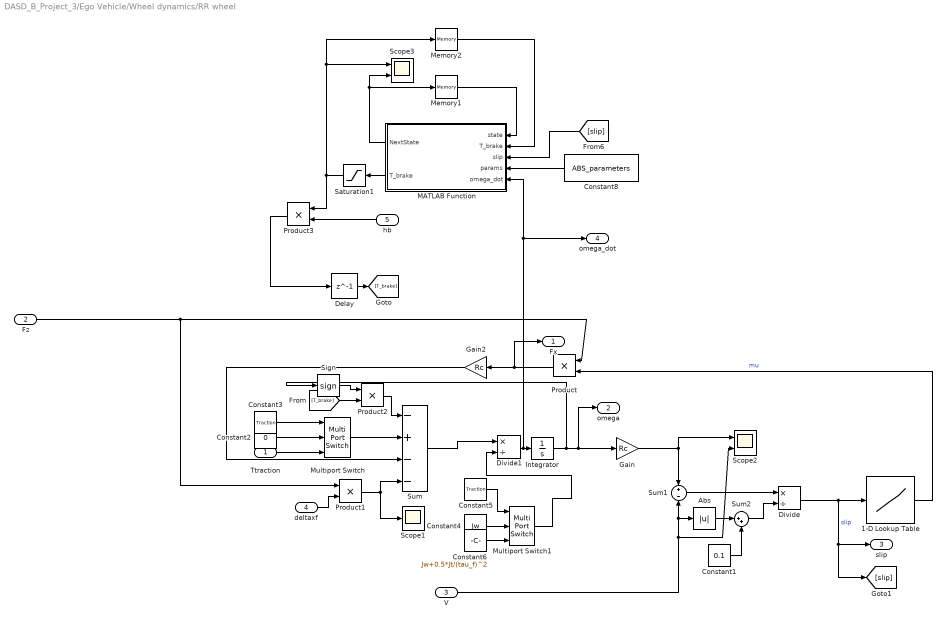
== system DASD_B_Project_3/Ego Vehicle/Wheel dynamics/RR wheel ==
  Ttraction : Inport
  Fz : Inport  Port=2
  V : Inport  Port=3
  deltaxf : Inport  Port=4
  hb : Inport  Port=5
  1-D Lookup Table : Lookup_n-D  NumberOfTableDimensions=1  BreakpointsForDimension1=sigma_vec  Table=mu_vec  InternalRulePriority=Speed  RndMeth=Simplest
  Abs : Abs  SaturateOnIntegerOverflow=off
  Constant1 : Constant  Value=0.1
  Constant2 : Constant  Value=0
  Constant3 : Constant  Value=Traction
  Constant4 : Constant  Value=Jw
  Constant5 : Constant  Value=Traction
  Constant6 : Constant  Value=Jw+0.5*Jt/(tau_f)^2
  Constant8 : Constant  Value=ABS_parameters
  Delay : Delay  DelayLength=1
  Divide : Product  Inputs=*/
  Divide1 : Product  Inputs=*/
  Gain : Gain  Gain=Rc
  Gain2 : Gain  Gain=Rc
  Integrator : Integrator  InitialCondition=omega0
  MATLAB Function : MATLAB Function  TreatAsAtomicUnit=on
  Memory1 : Memory  InitialCondition=1
  Memory2 : Memory
  Multiport Switch : MultiPortSwitch  Inputs=2  SaturateOnIntegerOverflow=off  InputSameDT=off
  Multiport Switch1 : MultiPortSwitch  Inputs=2  SaturateOnIntegerOverflow=off  InputSameDT=off
  Product{,1..3} (4 alike) : Product
  Saturation1 : Saturate  UpperLimit=1500  LowerLimit=0
  Scope1 : Scope
      settings: ActiveDisplayYMinimum=1.21613  ActiveDisplayYMaximum=10.98872  DataLoggingVariableName=ScopeData8
  Scope2 : Scope  NumInputPorts=2
      settings: ActiveDisplayYMinimum=-5.73063  ActiveDisplayYMaximum=50.63674  DataLoggingVariableName=ScopeData6
  Scope3 : Scope  NumInputPorts=2
      settings: ActiveDisplayYMinimum=-48.33125  ActiveDisplayYMaximum=435.48125  DataLoggingVariableName=ScopeData4
  Sign : Signum
  Sum : Sum  Inputs=-+--
  Sum1 : Sum  Inputs=+-
  Sum2 : Sum  Inputs=|++
  Fx : Outport
  omega : Outport  Port=2
  slip : Outport  Port=3
  omega_dot : Outport  Port=4
  wires:
  [T_brake] -> Product2/2
  Sign/1 -> Product2/1
  Product2/1 -> Sum/1
  Ttraction/1 -> Multiport Switch/3
  Constant2/1 -> Multiport Switch/2
  Constant4/1 -> Multiport Switch1/2
  Constant6/1 -> Multiport Switch1/3
  Sum/1 -> Divide1/1
  Multiport Switch1/1 -> Divide1/2
  Constant5/1 -> Multiport Switch1/1
  Constant3/1 -> Multiport Switch/1
  Multiport Switch/1 -> Sum/2
  Product1/1 -> Scope1/1, Sum/4
  deltaxf/1 -> Product1/2
  Constant1/1 -> Sum2/2
  Abs/1 -> Sum2/1
  Sum2/1 -> Divide/2
  Fz/1 -> Product1/1, Product/1
  Divide/1 -> [slip], slip/1, 1-D Lookup Table/1  "slip"
  Sum1/1 -> Divide/1
  Integrator/1 -> Gain/1, omega/1, Sign/1
  1-D Lookup Table/1 -> Product/2  "mu"
  Product/1 -> Gain2/1, Fx/1
  V/1 -> Scope2/2, Abs/1, Sum1/2
  Gain2/1 -> Sum/3
  Gain/1 -> Scope2/1, Sum1/1
  Divide1/1 -> MATLAB Function/5(omega_dot), omega_dot/1, Integrator/1
  Memory2/1 -> MATLAB Function/2("T_brake ")
  MATLAB Function/2(T_brake) -> Saturation1/1
  Constant8/1 -> MATLAB Function/4(params)
  Memory1/1 -> MATLAB Function/1(state)
  MATLAB Function/1(NextState) -> Memory1/1, Scope3/2
  [slip] -> MATLAB Function/3(slip)
  Saturation1/1 -> Memory2/1, Scope3/1, Product3/1
  Product3/1 -> Delay/1
  Delay/1 -> [T_brake]
  hb/1 -> Product3/2

== matlab function DASD_B_Project_3/Ego Vehicle/Wheel dynamics/FL wheel/MATLAB Function ==
  data: state input; T_brake input; slip input; params input; NextState output; omega_dot input; T_brake output
function [NextState, T_brake] = fcn(state, T_brake, slip, params, omega_dot)
%%% Next State represents the ABS valve condition at the next time step
%%% 1 = increase
%%% 2 = hold
%%% 3 = release
%%% 4 = hold
%%% 5 = increase
%%% 6 = hold
%%% 7 = increase less
%%% 8 = release (3)

lower_acc = params(1);
lower_slip = params(2);
higher_acc = params(3);
mean_acc = params(4);
rise_rate = params(5);
fall_rate = params(6);


switch state
    case 1
        if omega_dot < lower_acc
            NextState = 2;
        else
            NextState = 1;
        end
        T_brake = T_brake + rise_rate;
    case 2
        if slip < lower_slip
            NextState = 3;
        else
            NextState = 2;
        end
        T_brake = T_brake;
    case 3
        if slip > lower_slip
            NextState = 4;
        else
            NextState = 3;
        end
        T_brake = T_brake - fall_rate;
    case 4 
        if omega_dot > higher_acc
            NextState = 5;
        else
            NextState = 4;
        end
        T_brake = T_brake;
    case 5 
        if omega_dot < higher_acc
            NextState = 6;
        else
            NextState = 5;
        end
        T_brake = T_brake + rise_rate;
    case 6
        if omega_dot < mean_acc
            NextState = 7;
        else 
            NextState = 6;
        end
        T_brake = T_brake;
    case 7
        if omega_dot < lower_acc
            NextState = 3;
        else
            NextState = 7;
        end
        T_brake = T_brake + 0.5*rise_rate;
    otherwise
        NextState = state;
        T_brake = T_brake;
end
end
